simulink model "turbojet"  (R2018a)
settings: Solver=VariableStepAuto  StartTime=0.0  StopTime=0  RelTol=1e-3
libraries: motorlib x7
settings Model: Creator=mairon  LastModifiedBy=mairon

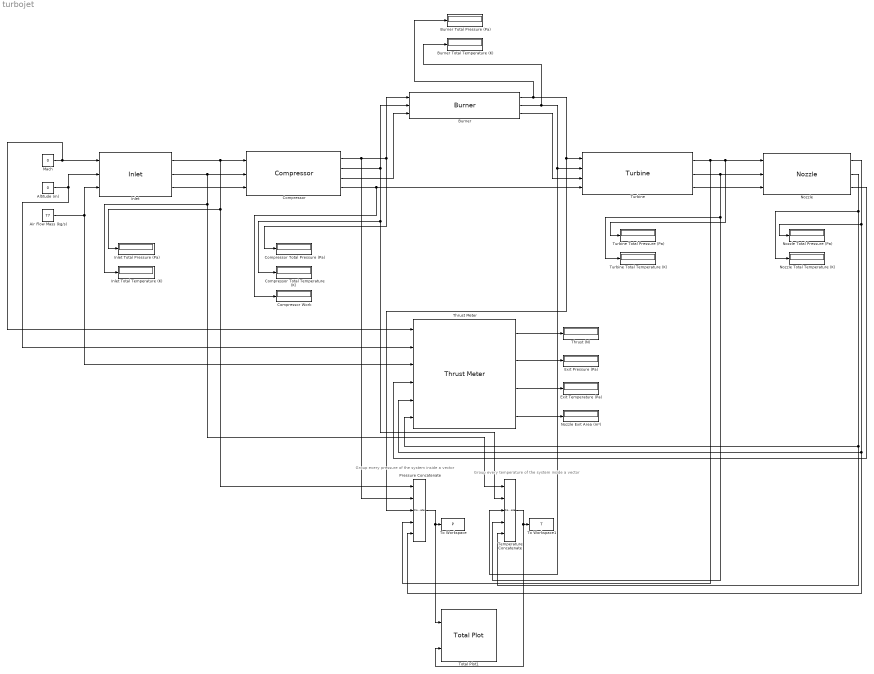
== system turbojet ==
  note: Group every temperature of the system inside a vector
  note: Group every pressure of the system inside a vector
  Air Flow Mass (kg/s) : Constant  Value=77
  Altitude (m) : Constant  Value=0
  Burner : motorlib/Burner
      settings: SourceProductName=Aeronautic Motor
  Burner Total Pressure (Pa) : Display
  Burner Total Temperature (K) : Display
  Compressor : motorlib/Compressor
      settings: SourceProductName=Aeronautic Motor
  Compressor Total Pressure (Pa) : Display
  Compressor Total Temperature (K) : Display
  Compressor Work : Display
  Exit Pressure (Pa) : Display
  Exit Temperature (Pa) : Display
  Inlet : motorlib/Inlet
      settings: SourceProductName=Aeronautic Motor
  Inlet Total Pressure (Pa) : Display
  Inlet Total Temperature (K) : Display
  Mach : Constant  Value=0
  Nozzle : motorlib/Nozzle
      settings: SourceProductName=Aeronautic Motor
  Nozzle Exit Area (m²) : Display
  "Nozzle Total Pressure (Pa) " : Display
  Nozzle Total Temperature (K) : Display
  Pressure Concatenate : Concatenate  NumInputs=5
  Temperature Concatenate : Concatenate  NumInputs=5
  Thrust (N) : Display
  Thrust Meter : motorlib/Thrust Meter
      settings: SourceProductName=Aeronautic Motor
  To Workspace : ToWorkspace  VariableName=P  SaveFormat=Timeseries  SampleTime=-1
  To Workspace1 : ToWorkspace  VariableName=T  SaveFormat=Timeseries  SampleTime=-1
  Total Plot1 : motorlib/Total Plot
      settings: SourceProductName=Stateflow  SourceProductBaseCode=SF
  Turbine : motorlib/Turbine
      settings: SourceProductName=Aeronautic Motor
  Turbine Total Pressure (Pa) : Display
  Turbine Total Temperature (K) : Display
  wires:
  Mach/1 -> Thrust Meter/1, Inlet/1
  Altitude (m)/1 -> Inlet/2, Thrust Meter/2
  Inlet/1 -> Inlet Total Pressure (Pa)/1, Pressure Concatenate/1, Compressor/1
  Air Flow Mass (kg/s)/1 -> Thrust Meter/3, Inlet/3
  Nozzle/1 -> Pressure Concatenate/5, Thrust Meter/5, "Nozzle Total Pressure (Pa) "/1
  Nozzle/2 -> Temperature Concatenate/5, Thrust Meter/6, Nozzle Total Temperature (K)/1
  Inlet/2 -> Temperature Concatenate/1, Inlet Total Temperature (K)/1, Compressor/2
  Inlet/3 -> Compressor/3
  Compressor/1 -> Pressure Concatenate/2, Burner/1, Compressor Total Pressure (Pa)/1
  Compressor/2 -> Burner/2, Temperature Concatenate/2, Compressor Total Temperature (K)/1
  Compressor/3 -> Burner/3
  Compressor/4 -> Compressor Work/1, Turbine/4
  Burner/1 -> Pressure Concatenate/3, Turbine/1, Burner Total Pressure (Pa)/1
  Burner/2 -> Temperature Concatenate/3, Turbine/2, Burner Total Temperature (K)/1
  Burner/3 -> Turbine/3
  Turbine/1 -> Pressure Concatenate/4, Nozzle/1, Turbine Total Pressure (Pa)/1
  Turbine/3 -> Nozzle/3
  Turbine/2 -> Temperature Concatenate/4, Turbine Total Temperature (K)/1, Nozzle/2
  Nozzle/3 -> Thrust Meter/4
  Thrust Meter/1 -> Thrust (N)/1
  Thrust Meter/2 -> Exit Pressure (Pa)/1
  Thrust Meter/3 -> Exit Temperature (Pa)/1
  Thrust Meter/4 -> Nozzle Exit Area (m²)/1
  Pressure Concatenate/1 -> Total Plot1/1, To Workspace/1
  Temperature Concatenate/1 -> Total Plot1/2, To Workspace1/1
